simulink model "1.-Simulador"  (R2023a)
settings: Solver=VariableStepAuto  StartTime=0.0  StopTime=0.01  RelTol=1e-3
settings Model: Creator=luisk  LastModifiedBy=luisk

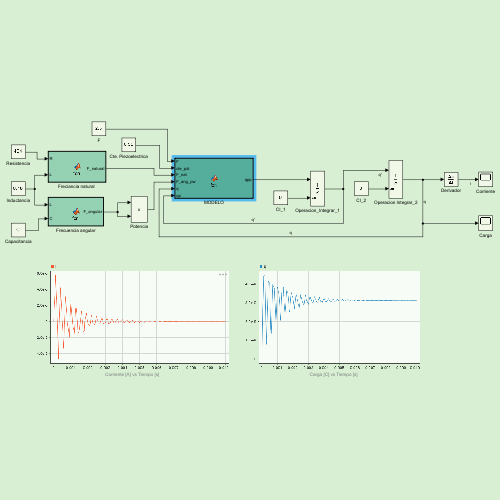
[thumbnail: Simulink's stored preview of the top-level diagram]
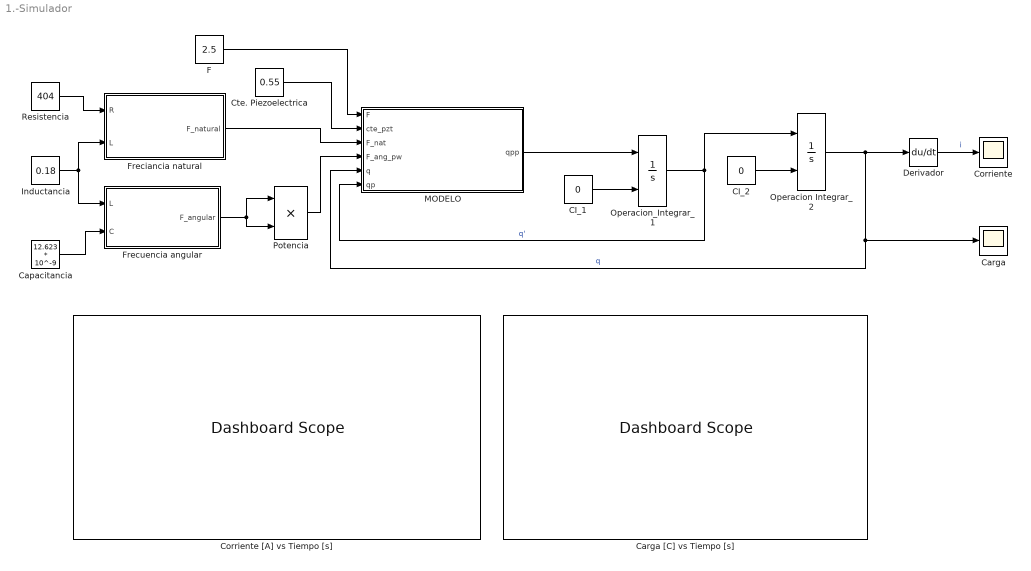
== system 1.-Simulador ==
  CI_1 : Constant  Value=0  SampleTime=0.0001
  CI_2 : Constant  Value=0  SampleTime=0.0001
  Capacitancia : Constant  Value=12.623 * 10^-9  SampleTime=0.0001
  Carga : Scope
  Carga [C] vs Tiempo [s] : DashboardScope
  Corriente : Scope
  Corriente [A] vs Tiempo [s] : DashboardScope
  Cte. Piezoelectrica : Constant  Value=0.55  SampleTime=0.0001
  Derivador : Derivative
  F : Constant  Value=2.5  SampleTime=0.0001
  "Freciancia natural " : MATLAB Function  TreatAsAtomicUnit=on
  Frecuencia angular : MATLAB Function  TreatAsAtomicUnit=on
  Inductancia : Constant  Value=0.18  SampleTime=0.0001
  MODELO : MATLAB Function  TreatAsAtomicUnit=on
  Operacion Integrar_2 : Integrator  InitialConditionSource=external
  Operacion_Integrar_1 : Integrator  InitialConditionSource=external
  Potencia : Product
  Resistencia : Constant  Value=404  SampleTime=0.0001
  wires:
  Resistencia/1 -> "Freciancia natural "/1(R)
  Inductancia/1 -> Frecuencia angular/1(L), "Freciancia natural "/2(L)
  Capacitancia/1 -> Frecuencia angular/2(C)
  Frecuencia angular/1(F_angular) -> Potencia/1, Potencia/2
  Potencia/1 -> MODELO/4(F_ang_pw)
  "Freciancia natural "/1(F_natural) -> MODELO/3(F_nat)
  Cte. Piezoelectrica/1 -> MODELO/2(cte_pzt)
  F/1 -> MODELO/1(F)
  MODELO/1(qpp) -> Operacion_Integrar_1/1
  Operacion_Integrar_1/1 -> Operacion Integrar_2/1, MODELO/6(qp)  "q'"
  Operacion Integrar_2/1 -> MODELO/5(q), Carga/1, Derivador/1  "q"
  Derivador/1 -> Corriente/1  "i"
  CI_1/1 -> Operacion_Integrar_1/2
  CI_2/1 -> Operacion Integrar_2/2

== matlab function 1.-Simulador/Frecuencia angular ==
  data: L input; F_angular output; C input
function F_angular = fcn(L, C)
F_angular = 1/sqrt(L*C);

== matlab function 1.-Simulador/Freciancia natural  ==
  data: R input; F_natural output; L input
function F_natural = fcn(R, L)
F_natural = R/(2*L);

== matlab function 1.-Simulador/MODELO ==
  data: F input; cte_pzt input; qpp output; F_nat input; F_ang_pw input; q input; qp input
function qpp = fcn(F, cte_pzt, F_nat, F_ang_pw, q, qp)
qpp = F*cte_pzt - 2 * F_nat * qp - F_ang_pw * q;
